simulink model "vehicle_par"  (R2017a)
settings: Solver=VariableStepAuto  StartTime=0.0  StopTime=200  RelTol=1e-3
undefined symbols (not defined in the file or in its folder): magnitude
libraries: elvio x19
settings Model: Creator=tstef  LastModifiedBy=tstef

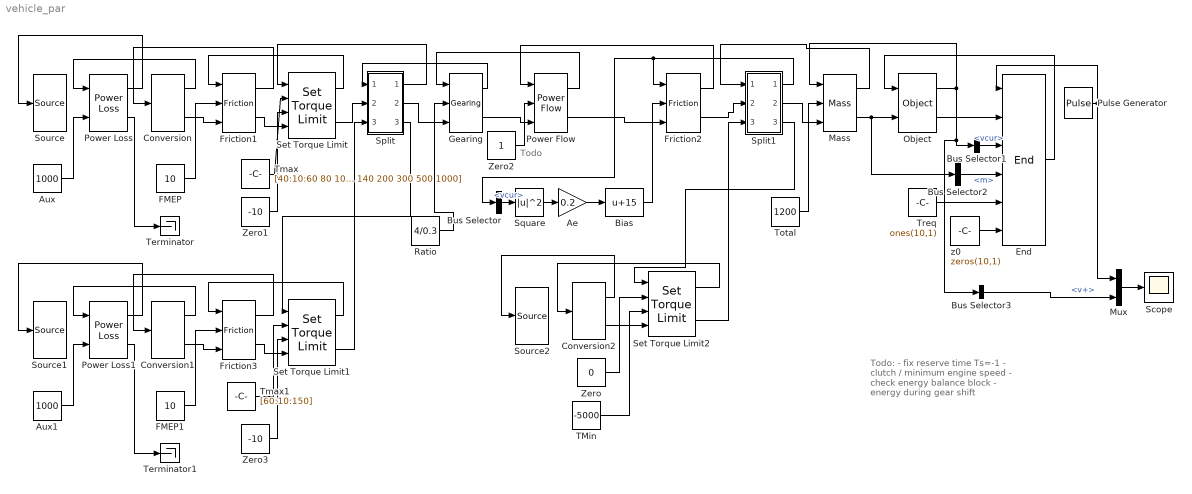
== system vehicle_par ==
  note: Todo:
      | - fix reserve time Ts=-1
      | - clutch / minimum engine speed
      | - check energy balance block
      | - energy during gear shift
  note: Todo
  Ae : Gain  Gain=0.2
  Aux : Constant  Value=1000
  Aux1 : Constant  Value=1000
  Bias : Bias  Bias=15
  Bus Selector : BusSelector  OutputSignals=vcur
  Bus Selector1 : BusSelector  OutputSignals=vcur
  Bus Selector2 : BusSelector  OutputSignals=m
  Bus Selector3 : BusSelector  OutputSignals=v+
  Conversion : elvio/Basics/Conversion
  Conversion1 : elvio/Basics/Conversion
  Conversion2 : elvio/Basics/Conversion
  End : elvio/Basics/End
  FMEP : Constant  Value=10
  FMEP1 : Constant  Value=10
  Friction1 : elvio/Basics/Friction
  Friction2 : elvio/Basics/Friction
  Friction3 : elvio/Basics/Friction
  Gearing : elvio/Basics/Gearing
  Mass : elvio/Basics/Mass
  Mux : Mux  Inputs=2
  Object : elvio/Basics/Object
  Power Flow : elvio/Basics/Power Flow
  Power Loss : elvio/Basics/Power Loss
  Power Loss1 : elvio/Basics/Power Loss
  Pulse Generator : DiscretePulseGenerator  PulseType=Time based  Amplitude=20  Period=100  PulseWidth=49.9
  Ratio : Constant  Value=4/0.3
  Scope : Scope
  Set Torque Limit : elvio/Basics/Set Torque Limit
  Set Torque Limit1 : elvio/Basics/Set Torque Limit
  Set Torque Limit2 : elvio/Basics/Set Torque Limit
  Source : elvio/Basics/Source
  Source1 : elvio/Basics/Source
  Source2 : elvio/Basics/Source
  Split : Subsystem
  Split1 : Subsystem
  Square : Math  Operator=magnitude^2  SaturateOnIntegerOverflow=on
  TMin : Constant  Value=-5000
  Terminator : Terminator
  Terminator1 : Terminator
  Tmax : Constant  Value=[40:10:60 80 100 140 200 300 500 1000]
  Tmax1 : Constant  Value=[60:10:150]
  Total : Constant  Value=1200
  Treq : Constant  Value=ones(10,1)
  Zero : Constant  Value=0
  Zero1 : Constant  Value=-10
  Zero2 : Constant
  Zero3 : Constant  Value=-10
  z0 : Constant  Value=zeros(10,1)
  wires:
  Friction2/2 -> Split1/2(F1)
  Gearing/2 -> Power Flow/3
  Set Torque Limit/2 -> Split/2(F1)
  Friction1/2 -> Set Torque Limit/4
  Conversion/2 -> Friction1/3
  Power Loss/1 -> Source/1
  Pulse Generator/1 -> End/1, Mux/1
  Conversion/1 -> Power Loss/1
  Friction1/1 -> Conversion/1
  Set Torque Limit/1 -> Friction1/1
  Split/1(v1) -> Set Torque Limit/1
  Friction2/1 -> Power Flow/1
  Split1/1(v1) -> Friction2/1, Bus Selector/1
  Object/1 -> Mass/1, Bus Selector3/1, Bus Selector1/1
  End/1 -> Object/1
  FMEP/1 -> Friction1/2
  Aux/1 -> Power Loss/2
  Tmax/1 -> Set Torque Limit/2
  Zero1/1 -> Set Torque Limit/3
  Ratio/1 -> Gearing/2
  Total/1 -> Mass/2
  Object/2 -> End/2
  Power Loss/2 -> Terminator/1
  Square/1 -> Ae/1
  Ae/1 -> Bias/1
  Bias/1 -> Friction2/2
  Bus Selector/1 -> Square/1  "<vcur>"
  Bus Selector1/1 -> End/3  "<vcur>"
  Mass/2 -> Bus Selector2/1, Object/2
  z0/1 -> End/6
  Treq/1 -> End/5
  Bus Selector2/1 -> End/4  "<m>"
  Power Flow/2 -> Friction2/3
  Power Flow/1 -> Gearing/1
  Zero2/1 -> Power Flow/2
  Split/2(F+) -> Gearing/3
  Power Loss1/2 -> Terminator1/1
  Zero3/1 -> Set Torque Limit1/3
  Tmax1/1 -> Set Torque Limit1/2
  Aux1/1 -> Power Loss1/2
  FMEP1/1 -> Friction3/2
  Split/3(v2) -> Set Torque Limit1/1
  Set Torque Limit1/1 -> Friction3/1
  Friction3/1 -> Conversion1/1
  Conversion1/1 -> Power Loss1/1
  Power Loss1/1 -> Source1/1
  Conversion1/2 -> Friction3/3
  Friction3/2 -> Set Torque Limit1/4
  Set Torque Limit1/2 -> Split/3(F2)
  Gearing/1 -> Split/1(v+)
  Split1/3(v2) -> Set Torque Limit2/1
  Mass/1 -> Split1/1(v+)
  Split1/2(F+) -> Mass/3
  Conversion2/1 -> Source2/1
  Set Torque Limit2/2 -> Split1/3(F2)
  Set Torque Limit2/1 -> Conversion2/1
  Conversion2/2 -> Set Torque Limit2/4
  Zero/1 -> Set Torque Limit2/2
  TMin/1 -> Set Torque Limit2/3
  Bus Selector3/1 -> Mux/2  "<v+>"
  Mux/1 -> Scope/1

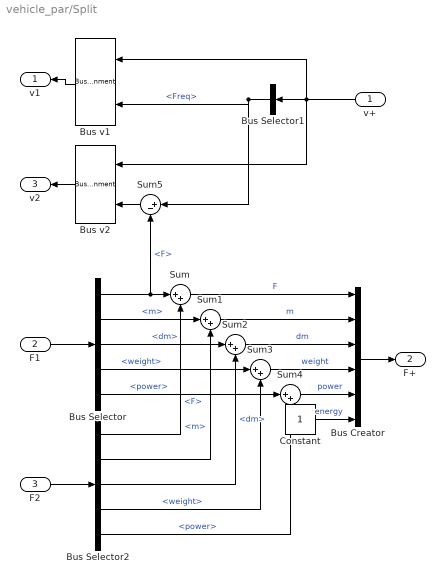
== system vehicle_par/Split ==
  v+ : Inport
  F1 : Inport  Port=2
  F2 : Inport  Port=3
  Bus Creator : BusCreator  Inputs=6
  Bus Selector : BusSelector  OutputSignals=F,m,dm,weight,power
  Bus Selector1 : BusSelector  OutputSignals=Freq
  Bus Selector2 : BusSelector  OutputSignals=F,m,dm,weight,power
  Bus v1 : BusAssignment  AssignedSignals=Freq
  Bus v2 : BusAssignment  AssignedSignals=Freq
  Constant : Constant
  Sum{,1..4} (5 alike) : Sum  Inputs=|++
  Sum5 : Sum  Inputs=|+-
  v1 : Outport
  F+ : Outport  Port=2
  v2 : Outport  Port=3
  wires:
  F1/1 -> Bus Selector/1
  Bus v1/1 -> v1/1
  Bus Selector1/1 -> Sum5/1, Bus v1/2  "<Freq>"
  Bus v2/1 -> v2/1
  v+/1 -> Bus v2/1, Bus v1/1, Bus Selector1/1
  Bus Selector/4 -> Sum3/1  "<weight>"
  Bus Selector/3 -> Sum2/1  "<dm>"
  Bus Selector/5 -> Sum4/1  "<power>"
  Bus Selector/2 -> Sum1/1  "<m>"
  Bus Selector/1 -> Sum5/2, Sum/1  "<F>"
  F2/1 -> Bus Selector2/1
  Bus Selector2/1 -> Sum/2  "<F>"
  Bus Selector2/2 -> Sum1/2  "<m>"
  Bus Selector2/3 -> Sum2/2  "<dm>"
  Bus Selector2/4 -> Sum3/2  "<weight>"
  Bus Selector2/5 -> Sum4/2  "<power>"
  Sum/1 -> Bus Creator/1  "F"
  Sum1/1 -> Bus Creator/2  "m"
  Sum2/1 -> Bus Creator/3  "dm"
  Sum3/1 -> Bus Creator/4  "weight"
  Sum4/1 -> Bus Creator/5  "power"
  Constant/1 -> Bus Creator/6  "energy"
  Bus Creator/1 -> F+/1
  Sum5/1 -> Bus v2/2

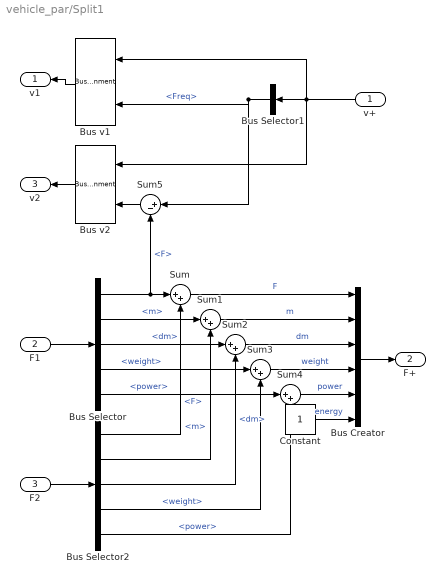
== system vehicle_par/Split1 ==
  v+ : Inport
  F1 : Inport  Port=2
  F2 : Inport  Port=3
  Bus Creator : BusCreator  Inputs=6
  Bus Selector : BusSelector  OutputSignals=F,m,dm,weight,power
  Bus Selector1 : BusSelector  OutputSignals=Freq
  Bus Selector2 : BusSelector  OutputSignals=F,m,dm,weight,power
  Bus v1 : BusAssignment  AssignedSignals=Freq
  Bus v2 : BusAssignment  AssignedSignals=Freq
  Constant : Constant
  Sum{,1..4} (5 alike) : Sum  Inputs=|++
  Sum5 : Sum  Inputs=|+-
  v1 : Outport
  F+ : Outport  Port=2
  v2 : Outport  Port=3
  wires:
  Sum5/1 -> Bus v2/2
  Bus Creator/1 -> F+/1
  Constant/1 -> Bus Creator/6  "energy"
  Sum4/1 -> Bus Creator/5  "power"
  Sum3/1 -> Bus Creator/4  "weight"
  Sum2/1 -> Bus Creator/3  "dm"
  Sum1/1 -> Bus Creator/2  "m"
  Sum/1 -> Bus Creator/1  "F"
  Bus Selector2/5 -> Sum4/2  "<power>"
  Bus Selector2/4 -> Sum3/2  "<weight>"
  Bus Selector2/3 -> Sum2/2  "<dm>"
  Bus Selector2/2 -> Sum1/2  "<m>"
  Bus Selector2/1 -> Sum/2  "<F>"
  F2/1 -> Bus Selector2/1
  Bus Selector/1 -> Sum/1, Sum5/2  "<F>"
  Bus Selector/2 -> Sum1/1  "<m>"
  Bus Selector/5 -> Sum4/1  "<power>"
  Bus Selector/3 -> Sum2/1  "<dm>"
  Bus Selector/4 -> Sum3/1  "<weight>"
  v+/1 -> Bus Selector1/1, Bus v1/1, Bus v2/1
  Bus v2/1 -> v2/1
  Bus Selector1/1 -> Bus v1/2, Sum5/1  "<Freq>"
  Bus v1/1 -> v1/1
  F1/1 -> Bus Selector/1
